simulink model "Road monito-2024r"  (R2021a)
settings: Solver=FixedStepDiscrete  StartTime=0.0  StopTime=inf  FixedStep=0.1  RelTol=1e-3
libraries: simulink x29
(part 1 of 2)
settings Model: Creator=lenovo  LastModifiedBy=lenovo
settings OptimizationCC: DefaultParameterBehavior=Inlined  EnhancedBackFolding=on  PassReuseOutputArgsAs=Individual arguments  ZeroExternalMemoryAtStartup=off  ZeroInternalMemoryAtStartup=off  OptimizeBlockOrder=speed  DifferentSizesBufferReuse=on  OptimizationCustomize=off  EfficientTunableParamExpr=on
settings DebuggingCC: ParameterTunabilityLossMsg=error
settings SFSimCC: MATLABDynamicMemAlloc=off
settings RTWCC: SystemTargetFile=ert.tlc  GenCodeOnly=on  PackageName=VM  TemplateMakefile=ert_default_tmf  GenerateReport=on  Toolchain=Microsoft Visual C++ 2019 v16.0 | nmake (64-bit Windows)  LaunchReport=on  TargetLang=C++
settings CodeAppCC: ForceParamTrailComments=on  IgnoreCustomStorageClasses=off  OperatorAnnotations=on  SimulinkDataObjDesc=on  SFDataObjDesc=on  InsertBlockDesc=on
settings ERTTargetCC: TargetLangStandard=C++03 (ISO)  GenerateSampleERTMain=on  CodeInterfacePackaging=C++ class  SupportContinuousTime=on  SupportVariableSizeSignals=on  InlinedParameterPlacement=NonHierarchical  RootIOFormat=Structure reference  ERTCustomFileTemplate=example_file_process.tlc

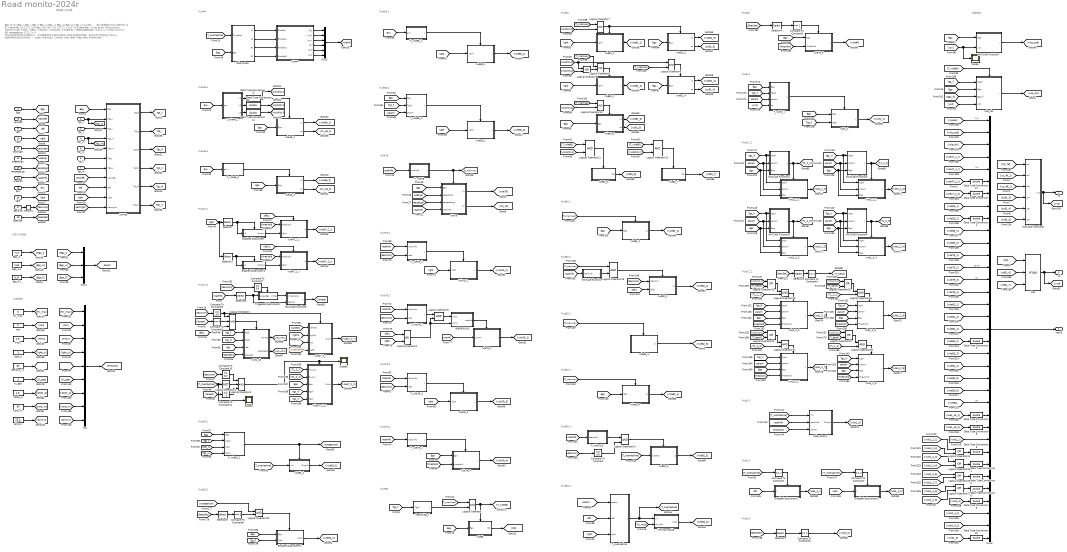
== system Road monito-2024r ==
  note: 法规阈值
  note: 自车几何参数
  note: Rule79.2
  note: Rule79.1
  note: Rule46.2
  note: 信息输入及处理
  note: Rule53.1
  note: Rule78
  note: Rule46.1
  note: Rule53.2
  note: Rule79.4
  note: Rule80
  note: Rule82.2
  note: Rule44
  note: Rule79.3
  note: Rule1.5
  note: Rule1.4
  note: Rule82.4
  note: Rule1.2.1
  note: Rule1.2.2
  note: Rule81
  note: Rule84
  note: Rule82.3
  note: Rule47.2
  note: Rule82.4
  note: Rule58.2
  note: Rule47.1
  note: Ego: [1 7]; [Ego_x Ego_y Ego_h Ego_vx Ego_vy Ego_ax Ego_ay]
      | Tgt_xx: [1 20]; 输入速度单位m/s
      | laneline: [1 6]; [identifier C3 C2 C1 C0 type] y = C3x^3 + C2x^2 + C1x +C0
      | identifier: -1(not exist) 0(Occlusion) 1(exist)
      | type: 1实线，2虚线，3双实线，4左实右虚，5左虚右实，6路肩
      | speedsign: [1 4]; [x y vxmax vxmin = 60]
      | respeedsign: [1 2]; [x y]
      | 自车坐标系原点位于后轴中心，所以需要自车长宽及后轴中心到自车前轴的距离；他车坐标为矩形的几何中心
      | roadinfo:[type,ID,Num]； type:1 mainway, 2 ramp, 3 acc lane, 4 dec lane, 5 eme lane
      | ID:自车所在的车道id，各类型均为最左侧车道id为1，往右递增；
      | Num:同类型同方向车道数
      | Env:[visibility, slip, night]；visibility能见度，slip高滑移路面标识符(1true，0false)，night夜间标识符
      | light:[left, right, fog, far, near, position, front, rear, waring] 均为标识符
      | decision:行为决策信息：1向左换道，2向右换道，3超车，4停车，5倒车，6掉头
      | SpecSec:[bend, tunnel, construction, diversion, merge, mergefollow]；
      | bend弯道路段，tunnel隧道路段，construction施工路段，diversion导流区域，merge合并路段区域，mergefollow合并路段后的区域；(overlap即为进入）
  note: Rule58.1
  note: 结果输出
  note: Rule82.1
  note: Rule82.6
  note: Rule1.3
  note: Rule1.1
  Ego : Inport  PortDimensions=[1 7]
  Tgt_x : Inport  Port=2  PortDimensions=[1 20]
  Tgt_y : Inport  Port=3  PortDimensions=[1 20]
  Tgt_vx : Inport  Port=4  PortDimensions=[1 20]
  Tgt_vy : Inport  Port=5  PortDimensions=[1 20]
  Tgt_l : Inport  Port=6  PortDimensions=[1 20]
  Tgt_w : Inport  Port=7  PortDimensions=[1 20]
  nextleft : Inport  Port=8  PortDimensions=[1 6]
  left : Inport  Port=9  PortDimensions=[1 6]
  right : Inport  Port=10  PortDimensions=[1 6]
  nextright : Inport  Port=11  PortDimensions=[1 6]
  speedsign : Inport  Port=12  PortDimensions=[1 4]
  respeedsign : Inport  Port=13  PortDimensions=[1 2]
  roadinfo : Inport  Port=14  PortDimensions=[1 3]
  Env : Inport  Port=15  PortDimensions=[1 3]
  light : Inport  Port=16  PortDimensions=[1 9]
  decision : Inport  Port=17  PortDimensions=[1 1]
  SpecSec : Inport  Port=18  PortDimensions=[1 6]
  Compare To Constant{,7..8,10} (4 alike) : simulink/Logic and Bit Operations/Compare To Constant  relop===  const=3.0  OutDataTypeStr=boolean
  Compare To Constant{1,3..6} (5 alike) : simulink/Logic and Bit Operations/Compare To Constant  relop===  const=1  OutDataTypeStr=boolean
  Compare To Constant11 : simulink/Logic and Bit Operations/Compare To Constant  relop===  const=-1  OutDataTypeStr=boolean
  Compare To Constant2 : simulink/Logic and Bit Operations/Compare To Constant  relop===  const=2  OutDataTypeStr=boolean
  Compare To Constant9 : simulink/Logic and Bit Operations/Compare To Constant  relop===  const=0  OutDataTypeStr=boolean
  Data Type Conversion{,1..14} (15 alike) : DataTypeConversion  OutDataTypeStr=double
  Ego_fl1 : Constant  Value=6.24
  Ego_l1 : Constant  Value=7.27
  Ego_w1 : Constant  Value=2.55
  Enabled Subsystem : Subsystem  TreatAsAtomicUnit=on
  Enabled Subsystem1 : Subsystem  TreatAsAtomicUnit=on
  Enabled Subsystem2 : Subsystem  TreatAsAtomicUnit=on
  Enabled Subsystem3 : Subsystem  TreatAsAtomicUnit=on
  Enabled Subsystem4 : Subsystem  TreatAsAtomicUnit=on
  Logical Operator{,5,7..18,23} (15 alike) : Logic  AllPortsSameDT=off  OutDataTypeStr=boolean
  Logical Operator1 : Logic  Inputs=3  AllPortsSameDT=off  OutDataTypeStr=boolean
  Logical Operator{2,6,19..22,24..27} (10 alike) : Logic  Operator=OR  AllPortsSameDT=off  OutDataTypeStr=boolean
  Logical Operator3 : Logic  Inputs=3  AllPortsSameDT=off  OutDataTypeStr=boolean
  Logical Operator4 : Logic  Operator=NOT  AllPortsSameDT=off  OutDataTypeStr=boolean
  MATLAB Function : MATLAB Function  TreatAsAtomicUnit=on
  MATLAB Function1 : MATLAB Function  TreatAsAtomicUnit=on
  MATLAB Function2 : MATLAB Function  TreatAsAtomicUnit=on
  MATLAB Function3 : MATLAB Function  TreatAsAtomicUnit=on
  MATLAB Function4 : MATLAB Function  TreatAsAtomicUnit=on
  MATLAB Function5 : MATLAB Function  TreatAsAtomicUnit=on
  MATLAB Function6 : MATLAB Function  TreatAsAtomicUnit=on
  MATLAB Function7 : MATLAB Function  TreatAsAtomicUnit=on
  Max : MinMax  Function=max  Inputs=3
  Memory : Memory
  Mux : Mux  Inputs=9
  Mux1 : Mux  Inputs=3
  Mux2 : Mux  Inputs=6
  Mux3 : Mux  Inputs=35
  Scope : Scope
  Scope2 : Scope
  Scope4 : Scope
  Selector : Selector  InputPortWidth=9  IndexOptions=Index vector (dialog)  Indices=[1]  OutputSizes=1
  Selector1 : Selector  InputPortWidth=9  IndexOptions=Index vector (dialog)  Indices=[2]  OutputSizes=1
  Selector2 : Selector  InputPortWidth=6  IndexOptions=Index vector (dialog)  Indices=[4]  OutputSizes=1
  Selector3 : Selector  InputPortWidth=6  IndexOptions=Index vector (dialog)  Indices=[1]  OutputSizes=1
  Selector4 : Selector  InputPortWidth=6  IndexOptions=Index vector (dialog)  Indices=[3]  OutputSizes=1
  Selector5 : Selector  InputPortWidth=6  IndexOptions=Index vector (dialog)  Indices=[5]  OutputSizes=1
  Selector6 : Selector  InputPortWidth=3  IndexOptions=Index vector (dialog)  Indices=[2]  OutputSizes=1
  Subsystem : Subsystem
  Subsystem2 : Subsystem
  TTCx : Constant  Value=1.8
  T_overlapline : MATLAB Function  TreatAsAtomicUnit=on
  T_rule1_1 : MATLAB Function  TreatAsAtomicUnit=on
  T_rule46_1 : MATLAB Function  TreatAsAtomicUnit=on
  T_rule46_2 : MATLAB Function  TreatAsAtomicUnit=on
  T_rule53_1 : MATLAB Function  TreatAsAtomicUnit=on
  T_rule58_1 : MATLAB Function  TreatAsAtomicUnit=on
  T_rule58_2 : MATLAB Function  TreatAsAtomicUnit=on
  T_rule78 : MATLAB Function  TreatAsAtomicUnit=on
  T_rule79_1 : MATLAB Function  TreatAsAtomicUnit=on
  T_rule79_2 : MATLAB Function  TreatAsAtomicUnit=on
  T_rule79_3 : MATLAB Function  TreatAsAtomicUnit=on
  T_rule79_4 : MATLAB Function  TreatAsAtomicUnit=on
  T_rule79_5 : MATLAB Function  TreatAsAtomicUnit=on
  Timing module : Subsystem
  Triggered Subsystem2 : Subsystem  TreatAsAtomicUnit=on
  cl_gap : Constant  Value=3
  cons_vx : Constant  Value=80
  dclmin : Constant  Value=[-3.4 13.6]
  declane_vx : Constant  Value=60
  isexistTgt_f : MATLAB Function  TreatAsAtomicUnit=on
  latdis_p : Constant  Value=1.8
  light_cl : Constant  Value=3
  nan : Constant  Value=0
  rule1_1 : Subsystem  TreatAsAtomicUnit=on
  rule1_2_1 : Subsystem  TreatAsAtomicUnit=on
  rule1_2_2 : Subsystem  TreatAsAtomicUnit=on
  rule1_2_3 : Subsystem  TreatAsAtomicUnit=on
  rule1_2_4 : Subsystem  TreatAsAtomicUnit=on
  rule1_2_5 : Subsystem  TreatAsAtomicUnit=on
  rule1_2_6 : Subsystem  TreatAsAtomicUnit=on
  rule1_2_7 : Subsystem  TreatAsAtomicUnit=on
  rule1_2_8 : Subsystem  TreatAsAtomicUnit=on
  rule1_43 : Subsystem  TreatAsAtomicUnit=on
  rule44 : Subsystem
  rule46_1 : Subsystem  TreatAsAtomicUnit=on
  rule46_2 : Subsystem  TreatAsAtomicUnit=on
  rule47_1_l : Subsystem  TreatAsAtomicUnit=on
  rule47_1_r : Subsystem  TreatAsAtomicUnit=on
  rule47_2_r : Subsystem  TreatAsAtomicUnit=on
  rule53_1 : Subsystem  TreatAsAtomicUnit=on
  rule58_1 : Subsystem  TreatAsAtomicUnit=on
  rule58_2 : Subsystem  TreatAsAtomicUnit=on
  rule78 : Subsystem  TreatAsAtomicUnit=on
  rule79_1 : Subsystem  TreatAsAtomicUnit=on
  rule79_2 : Subsystem  TreatAsAtomicUnit=on
  rule79_3 : Subsystem  TreatAsAtomicUnit=on
  rule79_4 : Subsystem  TreatAsAtomicUnit=on
  rule79_5 : Subsystem  TreatAsAtomicUnit=on
  rule80 : Subsystem  TreatAsAtomicUnit=on
  rule81_1 : Subsystem  TreatAsAtomicUnit=on
  rule81_2 : Subsystem  TreatAsAtomicUnit=on
  rule81_3 : Subsystem  TreatAsAtomicUnit=on
  rule81_4 : Subsystem  TreatAsAtomicUnit=on
  rule81_5 : Subsystem  TreatAsAtomicUnit=on
  rule81_6 : Subsystem  TreatAsAtomicUnit=on
  rule81_7 : Subsystem  TreatAsAtomicUnit=on
  rule82_1 : Subsystem  TreatAsAtomicUnit=on
  rule82_2 : Subsystem  TreatAsAtomicUnit=on
  rule82_3 : Subsystem  TreatAsAtomicUnit=on
  rule82_4 : Subsystem  TreatAsAtomicUnit=on
  rule82_5 : Subsystem  TreatAsAtomicUnit=on
  rule_47_2_2 : Subsystem  TreatAsAtomicUnit=on
  rule_dis : Subsystem  TreatAsAtomicUnit=on
  tcl_max : Constant  Value=6
  zoning : MATLAB Function  TreatAsAtomicUnit=on
  使能信号生成 : Subsystem
  result : Outport
  cs : Outport  Port=2
  cd : Outport  Port=3
  tag scope: Ego=global, Env=global, Tgt_f=global, Tgt_lf=global, Tgt_lr=global, Tgt_r=global, Tgt_rf=global, Tgt_rr=global, left=global, light=global, nextleft=global, nextright=global, param=global, respdsign=global, right=global, roadinfo=global, spdsign=global, threshold=global
  wires:
  [T_mainway] -> rule82_4/Enable
  Selector3/1 -> Compare To Constant4/1
  [rule47_1_l] -> Mux3/4
  Logical Operator24/1 -> Data Type Conversion3/1
  [roadinfo] -> Selector6/1
  [Ego] -> rule1_2_5/3(Ego)
  rule81_3/2(cs) -> [cs81_3]
  Ego_w1/1 -> [Ego_w]
  [T1_2_2] -> Logical Operator16/2
  rule81_1/1(y) -> [rule81_1]
  [T1_2_3] -> Logical Operator17/2
  rule1_2_1/1(y) -> [rule1_2_1]
  Logical Operator15/1 -> rule1_2_5/Enable
  [laneot] -> Compare To Constant11/1
  Data Type Conversion7/1 -> Mux3/25
  [rule1_2_3] -> Logical Operator24/2
  [Tgt_f] -> isexistTgt_f/1(Tgt_f)
  [T_mainway] -> Logical Operator9/2
  Enabled Subsystem4/1(Out2) -> [rule53_2]
  MATLAB Function5/1(y) -> [laneot]
  Tgt_vx/1 -> [Tgt_vx], zoning/4(Tgt_vx)
  rule47_1_r/1(y1) -> [rule47_1_r]
  TTCx/1 -> [TTCx]
  Selector4/1 -> Compare To Constant5/1
  Logical Operator19/1 -> Logical Operator15/1
  [Ego_l] -> Mux1/1
  [rule1_5] -> Data Type Conversion10/1
  [Ego_fl] -> Mux1/3
  [Visibility1] -> Logical Operator19/1
  T_rule1_1/1(y) -> rule1_1/Enable
  [rule_spd] -> Mux3/2
  [SpecSec] -> Selector2/1
  [light] -> rule81_1/1(light)
  [rule1_2_2] -> Logical Operator25/1
  Logical Operator21/1 -> Logical Operator17/1
  [nan] -> Mux/2
  Selector6/1 -> MATLAB Function5/2(laneid), Triggered Subsystem2/1(lane_Ego)
  Data Type Conversion6/1 -> Mux3/31
  T_rule79_5/1(y) -> Logical Operator14/1
  Enabled Subsystem3/1(y) -> [rule1_4_2]
  Logical Operator26/1 -> Data Type Conversion5/1
  [param] -> T_rule1_1/3(param)
  rule79_5/1(y) -> [rule84]
  rule81_5/1(y1) -> [rule81_5]
  [CD] -> Max/1
  Data Type Conversion10/1 -> Mux3/35
  [T_bend] -> Logical Operator20/2
  [rule81_1] -> Mux3/16
  Triggered Subsystem2/1(initial) -> MATLAB Function5/1(initiallane)
  nan/1 -> [nan]
  [T_bend] -> Logical Operator22/2
  [Ego] -> rule81_4/1(Ego)
  Compare To Constant2/1 -> Enabled Subsystem3/Enable
  [light] -> rule58_1/1(light)
  Subsystem/4(R2) -> rule44/4(Enable3)
  Logical Operator9/1 -> rule81_4/Enable
  rule82_2/1(y1) -> [rule82_2]
  Compare To Constant11/1 -> Logical Operator3/3
  Mux/1 -> [threshold]
  [T_overlapline] -> Subsystem2/1(In1)
  [left2] -> Logical Operator2/2
  [light] -> rule58_2/1(light)
  left/1 -> [left]
  [roadinfo] -> rule78/4(roadinfo)
  [rule1_43_1] -> Data Type Conversion7/1
  [threshold] -> Subsystem2/3(param)
  使能信号生成/1(enable) -> rule79_2/Enable
  [SpecSec] -> rule1_43/4(specsec)
  T_rule46_2/1(y) -> rule46_2/Enable
  rule46_1/1(y1) -> [rule46_1]
  Logical Operator7/1 -> rule81_3/Enable, rule81_1/Enable
  [threshold] -> rule1_2_8/4(threshold)
  rule79_1/1(y) -> [rule79_1]
  Mux3/1 -> result/1
  [rule53_2] -> Data Type Conversion1/1
  rule81_3/1(y1) -> [rule81_3]
  tcl_max/1 -> [Tcl_max]
  Data Type Conversion8/1 -> Mux3/26
  Tgt_w/1 -> zoning/7(Tgt_w)
  [Ego] -> rule1_2_6/3(Ego)
  Subsystem/1(L1) -> rule44/1(Enable)
  rule82_5/1(y1) -> [rule82_5]
  Logical Operator1/1 -> rule1_43/Enable
  [rule82_6] -> Mux3/23
  Enabled Subsystem1/1(Output) -> rule47_1_r/2(light)
  [decision] -> Compare To Constant7/1
  [light] -> rule79_1/1(light)
  rule1_2_2/1(y) -> [rule1_2_2]
  [CS_78] -> MATLAB Function6/1(cs1)
  [left1] -> Logical Operator1/3
  [Visibility1] -> Logical Operator21/1
  rule82_4/1(y1) -> [rule82_4]
  [threshold] -> rule47_1_r/1(threshold)
  [decision] -> Compare To Constant10/1
  Logical Operator22/1 -> Logical Operator18/1
  [Ego_w] -> Mux1/2
  [cd81_7] -> Max/3
  [Tgt_lf] -> rule1_43/2(Tgtlf)
  right/1 -> [right]
  [right] -> zoning/10(right)
  [Ego] -> T_rule1_1/1(Ego)
  [rule53_1] -> Mux3/8
  [Ego] -> rule81_5/1(Ego)
  [T_mainway] -> Logical Operator13/1
  [Ego] -> rule_dis/2(Ego)
  [cl_gap] -> Mux/6
  [Ego] -> rule82_1/1(Ego)
  [congestion] -> Logical Operator23/1
  [left] -> Enabled Subsystem2/1(u)
  Ego_fl1/1 -> [Ego_fl]
  Tgt_l/1 -> zoning/6(Tgt_l)
  [left] -> rule1_43/3(left)
  rule58_1/1(y) -> [rule58_1]
  T_overlapline/1(y) -> [T_overlapline], Timing module/1(y1)
  rule44/4(cl_f) -> Mux2/4
  rule47_1_l/1(y1) -> [rule47_1_l]
  rule58_2/1(y) -> [rule58_2]
  Logical Operator3/1 -> rule_47_2_2/Enable, Scope2/1
  [T_mainway] -> Logical Operator8/1
  [param] -> MATLAB Function4/2(param), rule1_2_4/2(param)
  [Visibility1] -> Logical Operator10/2
  zoning/4(Tgt_lr) -> [Tgt_lr]
  [cs81_4] -> MATLAB Function6/5(cs5)
  [light] -> rule79_3/1(light)
  [ycd] -> rule_dis/4(ycd)
  [Ego] -> rule1_2_2/3(Ego), MATLAB Function2/3(Ego)
  [threshold] -> rule79_4/2(threshold)
  [roadinfo] -> T_rule78/1(roadinfo)
  T_rule53_1/1(y) -> rule53_1/Enable, [congestion]
  Logical Operator10/1 -> rule81_5/Enable
  [T_overlapline] -> rule53_1/1(In1)
  [rule1_4_1] -> Mux3/33
  respeedsign/1 -> [respdsign]
  Mux1/1 -> [param]
  Logical Operator23/1 -> Enabled Subsystem4/Enable
  [T_mainway] -> Logical Operator/1
  rule44/3(cr_rr) -> Mux2/3
  [Tgt_rf] -> rule1_2_8/1(Tgtrr)
  [left1] -> rule47_2_r/4(left1)
  [T_mainway] -> Logical Operator10/1
  [declane_vx] -> Mux/5
  cl_gap/1 -> [cl_gap]
  [T_rule80] -> Logical Operator11/1
  [Ego] -> rule79_4/1(Ego)
  rule81_2/1(y) -> [rule81_2]
  [cs81_5] -> MATLAB Function6/6(cs6)
  [Ego] -> T_rule53_1/1(Ego)
  [Ego_fl] -> rule_dis/3(Ego_fl)
  [T1_2_4] -> Logical Operator18/2
  rule79_2/1(y) -> [rule79_2]
  speedsign/1 -> [spdsign]
  [roadinfo] -> MATLAB Function/1(roadinfo)
  zoning/3(Tgt_lf) -> [Tgt_lf]
  [rule44] -> Mux3/1  "1-6"
  [T_overlapline] -> Compare To Constant1/1
  [right] -> Enabled Subsystem3/1(u)
  [Ego] -> rule1_2_8/3(Ego)
  Logical Operator25/1 -> Data Type Conversion4/1
  nextleft/1 -> [nextleft]
  [rule1_2_6] -> Logical Operator27/1
  Compare To Constant10/1 -> Logical Operator3/1
  rule1_2_5/1(y) -> [rule1_2_5]
  [Tgt_rr] -> MATLAB Function4/1(Tgtrr), rule1_2_4/1(Tgtrr)
  rule79_3/1(y) -> [rule79_3]
  [rule79_3] -> Mux3/14  "20"
  Memory/1 -> [decision]
  [roadinfo] -> T_rule79_5/1(roadinfo)
  [rule1_4_2] -> Mux3/34
  [light_cl] -> Mux/4
  [param] -> rule1_2_8/2(param)
  rule78/2(y2) -> [CS_78]
  Logical Operator20/1 -> Logical Operator16/1
  [rule1_2_1] -> Logical Operator24/1
  [T1_2_1] -> Logical Operator15/2
  latdis_p/1 -> [latdis_p]
  decision/1 -> Memory/1
  [left] -> T_overlapline/2(left)
  Enabled Subsystem/1(Output) -> rule47_1_l/2(light)
  [Ego] -> rule1_1/1(Ego)
  [param] -> T_rule58_2/3(param)
  rule53_1/1(Output) -> [rule53_1]
  rule79_4/1(y) -> [rule79_4]
  Subsystem/3(R1) -> rule44/3(Enable2)
  [roadinfo] -> T_rule79_3/1(roadinfo)
  [Ego] -> MATLAB Function4/3(Ego), rule1_2_4/3(Ego)
  [TTCx] -> Mux/3
  Selector5/1 -> Compare To Constant6/1
  [T1_2_4] -> rule_47_2_2/2(t1_2_4)
  [Ego] -> rule46_1/1(Ego)
  rule81_4/1(y1) -> [rule81_4]
  [light] -> rule81_2/1(light)
  [decision] -> T_rule79_3/2(dec)
  [Visibility1] -> Logical Operator6/2
  [rule82_1] -> Mux3/18
  rule46_2/2(cs) -> [cs_46_2]
  [rule84] -> Mux3/24  "30"
  Compare To Constant7/1 -> Triggered Subsystem2/Trigger
  rule46_2/1(y1) -> [rule46_2]
  [Ego] -> zoning/1(Ego)
  Tgt_vy/1 -> zoning/5(Tgt_vy)
  T_rule58_1/1(y) -> rule58_1/Enable
  [rule82_2] -> Data Type Conversion2/1
  [T_rule80] -> rule_dis/Enable
  [Tgt_rf] -> rule1_2_2/1(Tgtrf), MATLAB Function2/1(Tgtrf)
  [nextleft] -> zoning/8(nextleft)
  [roadinfo] -> T_rule79_2/1(roadinfo)
  [rule1_2_7] -> Logical Operator26/2
  Enabled Subsystem2/1(y) -> [rule1_4_1]
  Tgt_x/1 -> [Tgt_x], zoning/2(Tgt_x)
  [cd81_6] -> Max/2
  [rule47_1_r] -> Mux3/5  "10"
  [T_overlapline] -> rule82_5/1(overlap)
  [respdsign] -> rule78/3(respeedsign)
  [T_bend] -> Logical Operator21/2
  [Tgt_x] -> T_rule53_1/3(Tgtx)
  [rule81_2] -> Mux3/17
  Logical Operator12/1 -> rule81_7/Enable
  Data Type Conversion9/1 -> Mux3/32
  [Tgt_rr] -> rule_47_2_2/5(Tgtrr)
  [rule82_3] -> Mux3/20
  Env/1 -> [Env]
  [cons_vx] -> Mux/8
  [param] -> rule1_2_3/2(param), MATLAB Function3/2(param)
  [rule58_1] -> Mux3/10
  [Tgt_rf] -> rule_47_2_2/4(Tgtrf)
  Data Type Conversion4/1 -> Mux3/29
  [rule79_1] -> Mux3/12
  [rule47_2_r] -> Data Type Conversion11/1
  [Tgt_vx] -> T_rule53_1/4(Tgtvx)
  [rule1_1] -> Mux3/27
  T_rule46_1/1(y1) -> Data Type Conversion12/1
  Timing module/1(Out2) -> [rule82_6]
  isexistTgt_f/1(y) -> Logical Operator/2
  rule78/1(y1) -> [rule78]
  MATLAB Function2/1(y) -> [T1_2_2], rule1_2_2/Enable
  [Tgt_f] -> rule_dis/1(Tgt_f)
  [Ego] -> rule1_2_1/3(Ego), MATLAB Function1/3(Ego)
  Selector/1 -> Enabled Subsystem/1(y1), Enabled Subsystem/Enable
  [right1] -> rule47_2_r/2(right1)
  [Tgt_f] -> rule1_1/2(Tgtf)
  [param] -> T_overlapline/1(param)
  [left1] -> rule82_2/2(left1)
  Logical Operator16/1 -> rule1_2_6/Enable
  [latdis_p] -> Mux/7
  [threshold] -> rule79_5/2(threshold)
  [Tgt_rf] -> rule1_2_6/1(Tgtrf)
  [param] -> rule1_2_7/2(param)
  [rule47_2_2] -> Data Type Conversion/1
  [Ego] -> rule79_5/1(Ego)
  declane_vx/1 -> [declane_vx]
  Logical Operator18/1 -> rule1_2_8/Enable
  T_rule79_2/1(y) -> Logical Operator5/1
  [Visibility1] -> Logical Operator22/1
  [param] -> rule1_2_6/2(param)
  MATLAB Function4/1(y) -> rule1_2_4/Enable, [T1_2_4]
  [Ego] -> rule1_2_3/3(Ego), MATLAB Function3/3(Ego)
  rule1_2_3/1(y) -> [rule1_2_3]
  zoning/1(Tgt_f) -> [Tgt_f]
  [T_bend] -> Logical Operator19/2
  [roadinfo] -> T_rule79_4/1(roadinfo)
  rule82_1/1(y1) -> [rule82_1]
  Logical Operator27/1 -> Data Type Conversion6/1
  [threshold] -> rule1_2_6/4(Threshold)
  Logical Operator5/1 -> 使能信号生成/1(pros)
  [Tgt_f] -> rule1_43/1(Tgtf)
  [Ego] -> T_rule58_2/1(Ego)
  [rule79_4] -> Mux3/15
  Compare To Constant3/1 -> [rule1_5]
  [param] -> rule1_2_2/2(param), MATLAB Function2/2(param)
  [Tgt_f] -> T_rule1_1/2(Tgt_f)
  rule80/1(CD) -> [CD]
  [Ego] -> rule_47_2_2/3(Ego)
  [SpecSec] -> Selector3/1
  rule46_1/2(cs) -> [cs_46_1]
  [right1] -> rule47_1_r/Enable
  Data Type Conversion/1 -> Mux3/7
  SpecSec/1 -> [SpecSec]
  Subsystem2/1(Output) -> [rule1_3]
  Data Type Conversion11/1 -> Mux3/6
  [rule1_2_8] -> Logical Operator27/2
  [rule58_2] -> Mux3/11
  [T_mainway] -> Logical Operator7/1
  Mux2/1 -> [rule44]
  zoning/5(Tgt_rf) -> [Tgt_rf]
  [Tgt_f] -> T_rule53_1/2(Tgt_f)
  [decision] -> T_rule79_1/2(dec)
  [decision] -> T_rule79_2/2(dec)
  roadinfo/1 -> [roadinfo]
  [T_overlapline] -> Compare To Constant2/1
  Logical Operator11/1 -> rule81_6/Enable
  [Ego] -> rule80/1(Ego)
  rule82_3/1(y1) -> [rule82_3]
  [left] -> zoning/9(left)
  Data Type Conversion3/1 -> Mux3/28
  Logical Operator/1 -> rule80/Enable, [T_rule80]
  rule1_1/1(y) -> [rule1_1]
  [T_overlapline] -> rule47_2_r/3(Tol)
  MATLAB Function3/1(y) -> rule1_2_3/Enable, [T1_2_3]
  [rule44] -> rule79_2/1(rule44)
  rule1_2_7/1(y) -> [rule1_2_7]
  [roadinfo] -> T_rule79_1/1(roadinfo)
  [threshold] -> rule1_2_5/4(threshold)
  rule47_2_r/1(Out1) -> [rule47_2_r]
  rule44/6(cl_lr) -> Mux2/6
  Tgt_y/1 -> zoning/3(Tgt_y)
  [Visibility3] -> Logical Operator11/2
  [Ego] -> rule46_2/1(Ego)
  [Tcl_max] -> Mux/1
  [rule1_2_5] -> Logical Operator26/1
  [T_overlapline] -> Scope4/1, Logical Operator4/1
  Logical Operator2/1 -> Logical Operator5/2, 使能信号生成/2(cons)
  zoning/6(Tgt_rr) -> [Tgt_rr]
  [threshold] -> rule1_2_7/4(threshold)
  T_rule79_1/1(y) -> rule79_1/Enable
  [right] -> T_overlapline/3(right)
  Ego_l1/1 -> [Ego_l]
  [decision] -> Compare To Constant8/1
  Logical Operator6/1 -> Logical Operator8/2
  light/1 -> [light]
  [rule82_4] -> Mux3/21
  [cs_46_1] -> MATLAB Function6/2(cs2)
  [light] -> Selector1/1, Selector/1
  T_rule79_3/1(y) -> rule79_3/Enable
  Subsystem/2(L2) -> rule44/2(Enable1)
  [T_overlapline] -> Subsystem/1(Toverlap)
  [rule79_2] -> Mux3/13  "18-19"
  Compare To Constant6/1 -> Logical Operator23/2
  [spdsign] -> rule78/2(speedsign)
  [Ego] -> Subsystem/2(Ego)
  Max/1 -> [ycd], cd/1
  [Ego] -> rule82_4/1(Ego)
  [decision] -> Compare To Constant/1
  MATLAB Function7/1(y) -> [rule_spd]
  MATLAB Function6/1(ycs) -> [ycs], cs/1
  [Env] -> T_rule46_1/1(env)
  MATLAB Function1/1(y) -> rule1_2_1/Enable, [T1_2_1]
  [laneot] -> rule47_2_r/1(laneot)
  [Visibility1] -> Logical Operator20/1
  [param] -> rule1_2_5/2(param)
  [T_mainway] -> rule82_1/Enable
  nextright/1 -> [nextright]
  Compare To Constant5/1 -> rule79_5/Enable
  rule1_2_8/1(y) -> [rule1_2_8]
  [Ego] -> rule1_2_7/3(Ego)
  Compare To Constant4/1 -> [T_bend]
  rule1_2_4/1(y) -> [rule1_2_4]
  Compare To Constant/1 -> Logical Operator14/2
  rule44/2(cr_rf) -> Mux2/2
  rule_47_2_2/1(Out1) -> [rule47_2_2]
  [rule1_43_2] -> Data Type Conversion8/1
  Data Type Conversion2/1 -> Mux3/19
  [Tgt_f] -> T_rule58_2/2(Tgt_f)
  Logical Operator13/1 -> rule82_2/Enable
  [cs81_3] -> MATLAB Function6/4(cs4)
  [Ego] -> Enabled Subsystem4/1(Ego)
  Logical Operator17/1 -> rule1_2_7/Enable
  [param] -> rule1_2_1/2(param), MATLAB Function1/2(param)
  MATLAB Function/1(y) -> Logical Operator13/2
  light_cl/1 -> [light_cl]
  zoning/2(Tgt_r) -> [Tgt_r]
  [rule82_5] -> Mux3/22
  [Tgt_lr] -> rule1_2_3/1(Tgtlr), MATLAB Function3/1(Tgtlr)
  [Visibility3] -> Logical Operator7/2
  T_rule78/1(y) -> [T_mainway], rule78/Enable
  [Tgt_lr] -> rule1_2_7/1(Tgtlr)
  [Visibility2] -> Logical Operator9/1, Logical Operator6/1
  [ycs] -> Scope/1, MATLAB Function7/2(ycs)
  [Tcl_max] -> Timing module/2(tcl_max)
  rule81_7/1(CD) -> [cd81_7]
  Selector1/1 -> Enabled Subsystem1/Enable, Enabled Subsystem1/1(y1)
  [rule1_3] -> Data Type Conversion9/1
  [Env] -> T_rule46_2/1(env)
  [T_mainway] -> rule82_3/Enable
  rule44/5(cl_lf) -> Mux2/5
  [rule1_2_4] -> Logical Operator25/2
  [Ego] -> MATLAB Function7/1(Ego)
  [Tgt_lf] -> rule1_2_1/1(Tgtlf), MATLAB Function1/1(Tgtlf)
  [cs_46_2] -> MATLAB Function6/3(cs3)
  rule81_6/1(CD) -> [cd81_6]
  [Visibility2] -> Logical Operator12/2
  rule44/1(cr_f) -> Mux2/1
  [T1_2_2] -> rule_47_2_2/1(T1_2_2)
  [roadinfo] -> Subsystem2/2(roadinfo)
  Data Type Conversion1/1 -> Mux3/9
  [SpecSec] -> Selector4/1
  Ego/1 -> [Ego]
  [left1] -> Logical Operator2/1
  Compare To Constant8/1 -> rule47_2_r/Enable, Logical Operator1/1
  rule1_43/2(specsecot) -> [rule1_43_2]
  rule1_2_6/1(y) -> [rule1_2_6]
  [Tgt_lf] -> rule1_2_5/1(Tgtlf)
  [decision] -> rule82_2/1(decision)
  Logical Operator4/1 -> Logical Operator3/2
  [Ego] -> rule81_3/1(Ego)
  rule81_5/2(cs) -> [cs81_5]
  [Tgt_f] -> Enabled Subsystem4/2(Tgtf)
  Compare To Constant9/1 -> Logical Operator1/2
  T_rule79_4/1(y) -> rule79_4/Enable
  [threshold] -> rule47_1_l/1(threshold)
  Compare To Constant1/1 -> Enabled Subsystem2/Enable
  [nextright] -> zoning/11(nextright)
  Data Type Conversion5/1 -> Mux3/30
  [Ego] -> rule78/1(Ego)
  rule_dis/1(y) -> [rule_dis]
  Logical Operator8/1 -> rule81_2/Enable
  Selector2/1 -> Compare To Constant3/1
  [rule_dis] -> Mux3/3
  [ycs] -> T_rule1_1/4(cs)
  [SpecSec] -> Selector5/1
  [left1] -> rule47_1_l/Enable
  cons_vx/1 -> [cons_vx]
  Logical Operator14/1 -> rule82_5/Enable
  rule1_43/1(frontot) -> [rule1_43_1]
  [Env] -> T_rule58_1/1(env)
  T_rule58_2/1(y) -> rule58_2/Enable
  [T_rule80] -> Logical Operator12/1
  [laneot] -> Compare To Constant9/1
  rule81_4/2(cs) -> [cs81_4]
  Data Type Conversion12/1 -> rule46_1/Enable, [Visibility1]
  T_rule46_1/2(y2) -> Data Type Conversion13/1
  Data Type Conversion13/1 -> [Visibility2]
  T_rule46_1/3(y3) -> Data Type Conversion14/1
  Data Type Conversion14/1 -> [Visibility3]
  dclmin/1 -> [dclmin]
  [dclmin] -> Mux/9

== system Road monito-2024r/Enabled Subsystem ==
  y1 : Inport
  Enable : EnablePort  StatesWhenEnabling=reset
  Add : Sum  Inputs=-+
  Clock3 : Clock
  Constant : Constant  Value=0
  Memory : Memory
  Memory1 : Memory
  Min : MinMax  Function=max  Inputs=2
  Triggered Subsystem2 : Subsystem  TreatAsAtomicUnit=on
  Output : Outport  OutputWhenDisabled=reset  InitialOutput=0
  wires:
  Clock3/1 -> Memory1/1
  y1/1 -> Memory/1
  Triggered Subsystem2/1(Output) -> Add/1
  Memory/1 -> Triggered Subsystem2/Trigger
  Memory1/1 -> Add/2, Triggered Subsystem2/1(In1)
  Min/1 -> Output/1
  Add/1 -> Min/1
  Constant/1 -> Min/2

== system Road monito-2024r/Enabled Subsystem1 ==
  y1 : Inport
  Enable : EnablePort  StatesWhenEnabling=reset
  Add : Sum  Inputs=-+
  Clock3 : Clock
  Constant : Constant  Value=0
  Memory : Memory
  Memory1 : Memory
  Min : MinMax  Function=max  Inputs=2
  Triggered Subsystem2 : Subsystem  TreatAsAtomicUnit=on
  Output : Outport  OutputWhenDisabled=reset  InitialOutput=0
  wires:
  Constant/1 -> Min/2
  Add/1 -> Min/1
  Min/1 -> Output/1
  Memory1/1 -> Triggered Subsystem2/1(In1), Add/2
  Memory/1 -> Triggered Subsystem2/Trigger
  Triggered Subsystem2/1(Output) -> Add/1
  y1/1 -> Memory/1
  Clock3/1 -> Memory1/1

== system Road monito-2024r/Enabled Subsystem2 ==
  u : Inport
  Enable : EnablePort
  MATLAB Function : MATLAB Function  TreatAsAtomicUnit=on
  y : Outport
  wires:
  u/1 -> MATLAB Function/1(left)
  MATLAB Function/1(y) -> y/1

== system Road monito-2024r/Enabled Subsystem3 ==
  u : Inport
  Enable : EnablePort
  MATLAB Function : MATLAB Function  TreatAsAtomicUnit=on
  y : Outport
  wires:
  u/1 -> MATLAB Function/1(left)
  MATLAB Function/1(y) -> y/1

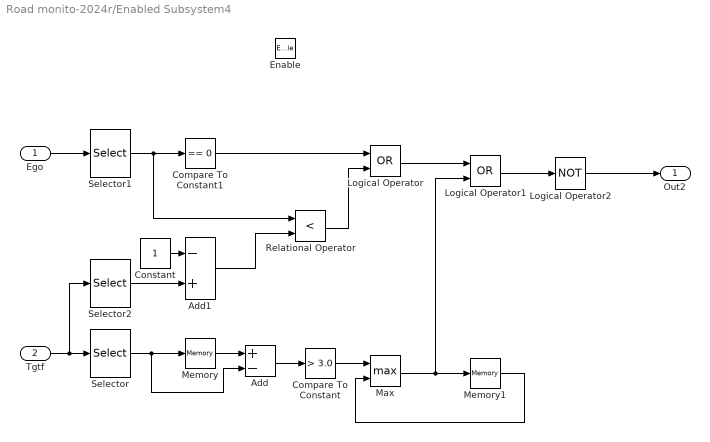
== system Road monito-2024r/Enabled Subsystem4 ==
  Ego : Inport
  Tgtf : Inport  Port=2
  Enable : EnablePort
  Add : Sum  Inputs=+-
  Add1 : Sum  Inputs=-+
  Compare To Constant : simulink/Logic and Bit Operations/Compare To Constant  relop=>  const=3.0  OutDataTypeStr=boolean
  Compare To Constant1 : simulink/Logic and Bit Operations/Compare To Constant  relop===  const=0  OutDataTypeStr=boolean
  Constant : Constant
  Logical Operator : Logic  Operator=OR  AllPortsSameDT=off  OutDataTypeStr=boolean
  Logical Operator1 : Logic  Operator=OR  AllPortsSameDT=off  OutDataTypeStr=boolean
  Logical Operator2 : Logic  Operator=NOT  AllPortsSameDT=off  OutDataTypeStr=boolean
  Max : MinMax  Function=max  Inputs=2
  Memory : Memory  InheritSampleTime=on
  Memory1 : Memory
  Relational Operator : RelationalOperator  Operator=<  OutDataTypeStr=boolean  RndMeth=Simplest
  Selector : Selector  InputPortWidth=6  IndexOptions=Index vector (dialog)  Indices=[1]  OutputSizes=1
  Selector1 : Selector  InputPortWidth=7  IndexOptions=Index vector (dialog)  Indices=[4]  OutputSizes=1
  Selector2 : Selector  InputPortWidth=6  IndexOptions=Index vector (dialog)  Indices=[3]  OutputSizes=1
  Out2 : Outport
  wires:
  Selector/1 -> Add/2, Memory/1
  Add/1 -> Compare To Constant/1
  Memory/1 -> Add/1
  Tgtf/1 -> Selector2/1, Selector/1
  Memory1/1 -> Max/2
  Max/1 -> Logical Operator1/2, Memory1/1
  Compare To Constant/1 -> Max/1
  Ego/1 -> Selector1/1
  Selector1/1 -> Relational Operator/1, Compare To Constant1/1
  Selector2/1 -> Add1/2
  Constant/1 -> Add1/1
  Add1/1 -> Relational Operator/2
  Compare To Constant1/1 -> Logical Operator/1
  Relational Operator/1 -> Logical Operator/2
  Logical Operator/1 -> Logical Operator1/1
  Logical Operator1/1 -> Logical Operator2/1
  Logical Operator2/1 -> Out2/1

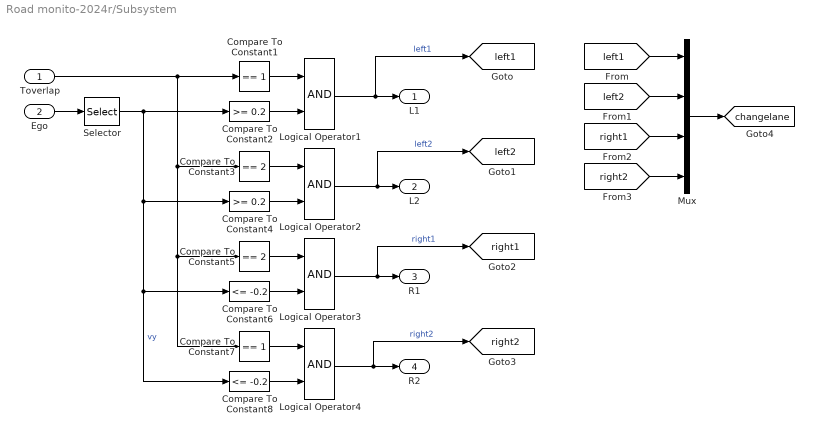
== system Road monito-2024r/Subsystem ==
  Toverlap : Inport
  Ego : Inport  Port=2
  Compare To Constant1 : simulink/Logic and Bit Operations/Compare To Constant  relop===  const=1  OutDataTypeStr=boolean
  Compare To Constant2 : simulink/Logic and Bit Operations/Compare To Constant  relop=>=  const=0.2  OutDataTypeStr=boolean
  Compare To Constant3 : simulink/Logic and Bit Operations/Compare To Constant  relop===  const=2  OutDataTypeStr=boolean
  Compare To Constant4 : simulink/Logic and Bit Operations/Compare To Constant  relop=>=  const=0.2  OutDataTypeStr=boolean
  Compare To Constant5 : simulink/Logic and Bit Operations/Compare To Constant  relop===  const=2  OutDataTypeStr=boolean
  Compare To Constant6 : simulink/Logic and Bit Operations/Compare To Constant  relop=<=  const=-0.2  OutDataTypeStr=boolean
  Compare To Constant7 : simulink/Logic and Bit Operations/Compare To Constant  relop===  const=1  OutDataTypeStr=boolean
  Compare To Constant8 : simulink/Logic and Bit Operations/Compare To Constant  relop=<=  const=-0.2  OutDataTypeStr=boolean
  Logical Operator{1..4} (4 alike) : Logic  AllPortsSameDT=off  OutDataTypeStr=boolean
  Mux : Mux
  Selector : Selector  InputPortWidth=7  IndexOptions=Index vector (dialog)  Indices=[5]  OutputSizes=1
  L1 : Outport
  L2 : Outport  Port=2
  R1 : Outport  Port=3
  R2 : Outport  Port=4
  tag scope: changelane=global, left1=global, left2=global, right1=global, right2=global
  wires:
  Toverlap/1 -> Compare To Constant7/1, Compare To Constant5/1, Compare To Constant3/1, Compare To Constant1/1
  Selector/1 -> Compare To Constant4/1, Compare To Constant8/1, Compare To Constant6/1, Compare To Constant2/1  "vy"
  Compare To Constant1/1 -> Logical Operator1/1
  Logical Operator1/1 -> [left1], L1/1  "left1"
  Compare To Constant2/1 -> Logical Operator1/2
  Ego/1 -> Selector/1
  Logical Operator2/1 -> [left2], L2/1  "left2"
  Compare To Constant3/1 -> Logical Operator2/1
  Compare To Constant4/1 -> Logical Operator2/2
  Logical Operator3/1 -> [right1], R1/1  "right1"
  Compare To Constant5/1 -> Logical Operator3/1
  Compare To Constant6/1 -> Logical Operator3/2
  Logical Operator4/1 -> [right2], R2/1  "right2"
  Compare To Constant7/1 -> Logical Operator4/1
  Compare To Constant8/1 -> Logical Operator4/2
  [left1] -> Mux/1
  [left2] -> Mux/2
  [right1] -> Mux/3
  [right2] -> Mux/4
  Mux/1 -> [changelane]

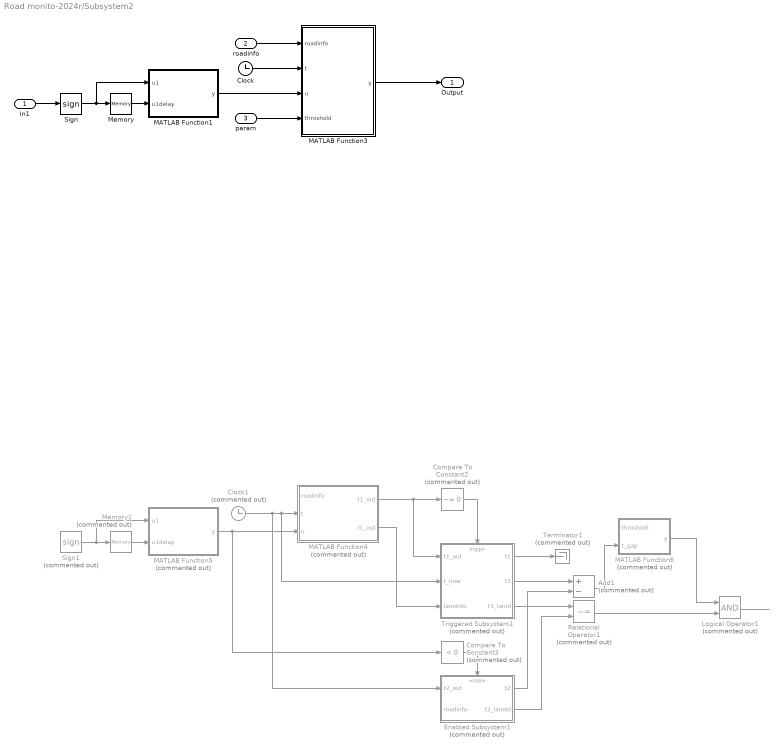
== system Road monito-2024r/Subsystem2 ==
  In1 : Inport
  roadinfo : Inport  Port=2
  param : Inport  Port=3
  Add1 : Sum  Commented=on  Inputs=+-
  Clock : Clock
  Clock1 : Clock  Commented=on
  Compare To Constant2 : simulink/Logic and Bit Operations/Compare To Constant  Commented=on  relop=~=  const=0  OutDataTypeStr=boolean
  Compare To Constant3 : simulink/Logic and Bit Operations/Compare To Constant  Commented=on  relop=<  const=0  OutDataTypeStr=boolean
  Enabled Subsystem1 : Subsystem  Commented=on  TreatAsAtomicUnit=on
  Logical Operator1 : Logic  Commented=on  AllPortsSameDT=off  OutDataTypeStr=boolean
  MATLAB Function1 : MATLAB Function  TreatAsAtomicUnit=on
  MATLAB Function3 : MATLAB Function  TreatAsAtomicUnit=on
  MATLAB Function4 : MATLAB Function  Commented=on  TreatAsAtomicUnit=on
  MATLAB Function5 : MATLAB Function  Commented=on  TreatAsAtomicUnit=on
  MATLAB Function6 : MATLAB Function  Commented=on  TreatAsAtomicUnit=on
  Memory : Memory
  Memory1 : Memory  Commented=on
  Relational Operator1 : RelationalOperator  Commented=on  Operator=~=  OutDataTypeStr=boolean  RndMeth=Simplest
  Sign : Signum
  Sign1 : Signum  Commented=on
  Terminator1 : Terminator  Commented=on
  Triggered Subsystem1 : Subsystem  Commented=on  TreatAsAtomicUnit=on
  Output : Outport
  wires:
  Clock/1 -> MATLAB Function3/2(t)
  Memory/1 -> MATLAB Function1/2(u1delay)
  Sign/1 -> MATLAB Function1/1(u1), Memory/1
  MATLAB Function1/1(y) -> MATLAB Function3/3(u)
  roadinfo/1 -> MATLAB Function3/1(roadinfo)
  In1/1 -> Sign/1
  param/1 -> MATLAB Function3/4(throshold)
  Relational Operator1/1 -> Logical Operator1/2
  Triggered Subsystem1/2(t3) -> Add1/1
  Enabled Subsystem1/2(t2_laneid) -> Relational Operator1/2
  Compare To Constant2/1 -> Triggered Subsystem1/Trigger
  Add1/1 -> MATLAB Function6/2(t_gap)
  MATLAB Function6/1(y) -> Logical Operator1/1
  MATLAB Function4/1(t1_out) -> Triggered Subsystem1/1(t1_out), Compare To Constant2/1
  Logical Operator1/1 -> ?
  Triggered Subsystem1/3(t1_lanid) -> Relational Operator1/1
  MATLAB Function4/2(l1_out) -> Triggered Subsystem1/3(laneinfo)
  Triggered Subsystem1/1(t1) -> Terminator1/1
  MATLAB Function5/1(y) -> MATLAB Function4/3(u), Compare To Constant3/1
  Memory1/1 -> MATLAB Function5/2(u1delay)
  Clock1/1 -> Enabled Subsystem1/1(t2_out), Triggered Subsystem1/2(t_now), MATLAB Function4/2(t)
  Compare To Constant3/1 -> Enabled Subsystem1/Enable
  Sign1/1 -> MATLAB Function5/1(u1), Memory1/1
  Enabled Subsystem1/1(t2) -> Add1/2
  MATLAB Function3/1(y) -> Output/1

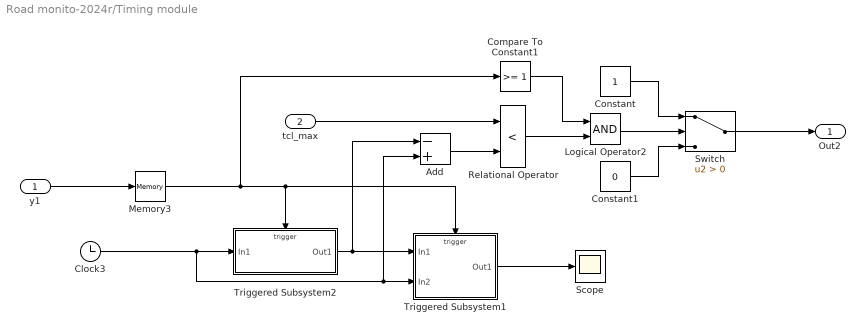
== system Road monito-2024r/Timing module ==
  y1 : Inport
  tcl_max : Inport  Port=2
  Add : Sum  Inputs=-+
  Clock3 : Clock
  Compare To Constant1 : simulink/Logic and Bit Operations/Compare To Constant  relop=>=  const=1  OutDataTypeStr=boolean
  Constant : Constant
  Constant1 : Constant  Value=0
  Logical Operator2 : Logic  AllPortsSameDT=off  OutDataTypeStr=boolean
  Memory3 : Memory
  Relational Operator : RelationalOperator  Operator=<  OutDataTypeStr=boolean  RndMeth=Simplest
  Scope : Scope
  Switch : Switch  Criteria=u2 > Threshold
  Triggered Subsystem1 : Subsystem  TreatAsAtomicUnit=on
  Triggered Subsystem2 : Subsystem  TreatAsAtomicUnit=on
  Out2 : Outport  VectorParamsAs1DForOutWhenUnconnected=off
  wires:
  Relational Operator/1 -> Logical Operator2/2
  Compare To Constant1/1 -> Logical Operator2/1
  Triggered Subsystem1/1(Out1) -> Scope/1
  Logical Operator2/1 -> Switch/2
  y1/1 -> Memory3/1
  Memory3/1 -> Compare To Constant1/1, Triggered Subsystem1/Trigger, Triggered Subsystem2/Trigger
  Add/1 -> Relational Operator/2
  Clock3/1 -> Add/2, Triggered Subsystem1/2(In2), Triggered Subsystem2/1(In1)
  Triggered Subsystem2/1(Out1) -> Add/1, Triggered Subsystem1/1(In1)
  tcl_max/1 -> Relational Operator/1
  Constant/1 -> Switch/1
  Constant1/1 -> Switch/3
  Switch/1 -> Out2/1

== system Road monito-2024r/Triggered Subsystem2 ==
  lane_Ego : Inport
  Trigger : TriggerPort  VariantControl=Variant
  initial : Outport  InitialOutput=0  VectorParamsAs1DForOutWhenUnconnected=off
  wires:
  lane_Ego/1 -> initial/1

== system Road monito-2024r/rule1_1 ==
  Ego : Inport
  Tgtf : Inport  Port=2
  Enable : EnablePort  StatesWhenEnabling=reset
  speed consistent : MATLAB Function  TreatAsAtomicUnit=on
  y : Outport  OutputWhenDisabled=reset  InitialOutput=0
  wires:
  Ego/1 -> speed consistent/1(Ego)
  speed consistent/1(y) -> y/1
  Tgtf/1 -> speed consistent/2(Tgtf)

== system Road monito-2024r/rule1_2_1 ==
  Tgtlf : Inport
  param : Inport  Port=2
  Ego : Inport  Port=3
  Enable : EnablePort  StatesWhenEnabling=reset
  LatDis : MATLAB Function  TreatAsAtomicUnit=on
  y : Outport  OutputWhenDisabled=reset  InitialOutput=0
  wires:
  LatDis/1(y) -> y/1
  Tgtlf/1 -> LatDis/1(Tgtlf)
  Ego/1 -> LatDis/3(Ego)
  param/1 -> LatDis/2(param)

== system Road monito-2024r/rule1_2_2 ==
  Tgtrf : Inport
  param : Inport  Port=2
  Ego : Inport  Port=3
  Enable : EnablePort  StatesWhenEnabling=reset
  LatDis : MATLAB Function  TreatAsAtomicUnit=on
  y : Outport  OutputWhenDisabled=reset  InitialOutput=0
  wires:
  LatDis/1(y) -> y/1
  Tgtrf/1 -> LatDis/1(Tgtrf)
  Ego/1 -> LatDis/3(Ego)
  param/1 -> LatDis/2(param)

== system Road monito-2024r/rule1_2_3 ==
  Tgtlr : Inport
  param : Inport  Port=2
  Ego : Inport  Port=3
  Enable : EnablePort  StatesWhenEnabling=reset
  LatDis : MATLAB Function  TreatAsAtomicUnit=on
  y : Outport  OutputWhenDisabled=reset  InitialOutput=0
  wires:
  LatDis/1(y) -> y/1
  Tgtlr/1 -> LatDis/1(Tgtlr)
  Ego/1 -> LatDis/3(Ego)
  param/1 -> LatDis/2(param)

== system Road monito-2024r/rule1_2_4 ==
  Tgtrr : Inport
  param : Inport  Port=2
  Ego : Inport  Port=3
  Enable : EnablePort  StatesWhenEnabling=reset
  LatDis : MATLAB Function  TreatAsAtomicUnit=on
  y : Outport  OutputWhenDisabled=reset  InitialOutput=0
  wires:
  LatDis/1(y) -> y/1
  Tgtrr/1 -> LatDis/1(Tgtrr)
  Ego/1 -> LatDis/3(Ego)
  param/1 -> LatDis/2(param)

== system Road monito-2024r/rule1_2_5 ==
  Tgtlf : Inport
  param : Inport  Port=2
  Ego : Inport  Port=3
  threshold : Inport  Port=4
  Enable : EnablePort  StatesWhenEnabling=reset
  LatDis : MATLAB Function  TreatAsAtomicUnit=on
  y : Outport  OutputWhenDisabled=reset  InitialOutput=0
  wires:
  LatDis/1(y) -> y/1
  Tgtlf/1 -> LatDis/1(Tgtlf)
  Ego/1 -> LatDis/3(Ego)
  param/1 -> LatDis/2(param)
  threshold/1 -> LatDis/4(threshlod)

== system Road monito-2024r/rule1_2_6 ==
  Tgtrf : Inport
  param : Inport  Port=2
  Ego : Inport  Port=3
  Threshold : Inport  Port=4
  Enable : EnablePort  StatesWhenEnabling=reset
  LatDis : MATLAB Function  TreatAsAtomicUnit=on
  y : Outport  OutputWhenDisabled=reset  InitialOutput=0
  wires:
  LatDis/1(y) -> y/1
  Tgtrf/1 -> LatDis/1(Tgtrf)
  Ego/1 -> LatDis/3(Ego)
  param/1 -> LatDis/2(param)
  Threshold/1 -> LatDis/4(threshlod)

== system Road monito-2024r/rule1_2_7 ==
  Tgtlr : Inport
  param : Inport  Port=2
  Ego : Inport  Port=3
  threshold : Inport  Port=4
  Enable : EnablePort  StatesWhenEnabling=reset
  LatDis : MATLAB Function  TreatAsAtomicUnit=on
  y : Outport  OutputWhenDisabled=reset  InitialOutput=0
  wires:
  LatDis/1(y) -> y/1
  Tgtlr/1 -> LatDis/1(Tgtlr)
  Ego/1 -> LatDis/3(Ego)
  param/1 -> LatDis/2(param)
  threshold/1 -> LatDis/4(threshlod)

== system Road monito-2024r/rule1_2_8 ==
  Tgtrr : Inport
  param : Inport  Port=2
  Ego : Inport  Port=3
  threshold : Inport  Port=4
  Enable : EnablePort  StatesWhenEnabling=reset
  LatDis : MATLAB Function  TreatAsAtomicUnit=on
  y : Outport  OutputWhenDisabled=reset  InitialOutput=0
  wires:
  LatDis/1(y) -> y/1
  Tgtrr/1 -> LatDis/1(Tgtrr)
  Ego/1 -> LatDis/3(Ego)
  param/1 -> LatDis/2(param)
  threshold/1 -> LatDis/4(threshlod)

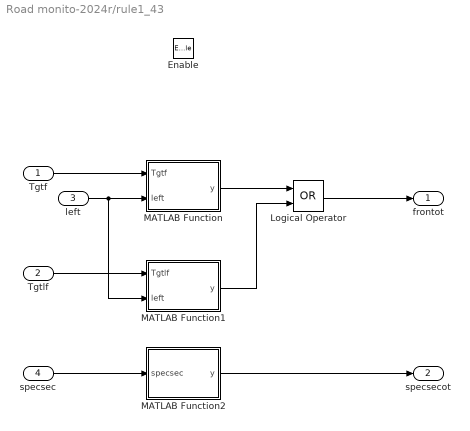
== system Road monito-2024r/rule1_43 ==
  Tgtf : Inport
  Tgtlf : Inport  Port=2
  left : Inport  Port=3
  specsec : Inport  Port=4
  Enable : EnablePort  StatesWhenEnabling=reset
  Logical Operator : Logic  Operator=OR  AllPortsSameDT=off  OutDataTypeStr=boolean
  MATLAB Function : MATLAB Function  TreatAsAtomicUnit=on
  MATLAB Function1 : MATLAB Function  TreatAsAtomicUnit=on
  MATLAB Function2 : MATLAB Function  TreatAsAtomicUnit=on
  frontot : Outport  OutputWhenDisabled=reset  InitialOutput=0
  specsecot : Outport  Port=2  OutputWhenDisabled=reset  InitialOutput=0
  wires:
  Tgtf/1 -> MATLAB Function/1(Tgtf)
  MATLAB Function/1(y) -> Logical Operator/1
  MATLAB Function1/1(y) -> Logical Operator/2
  Logical Operator/1 -> frontot/1
  Tgtlf/1 -> MATLAB Function1/1(Tgtlf)
  left/1 -> MATLAB Function1/2(left), MATLAB Function/2(left)
  specsec/1 -> MATLAB Function2/1(specsec)
  MATLAB Function2/1(y) -> specsecot/1

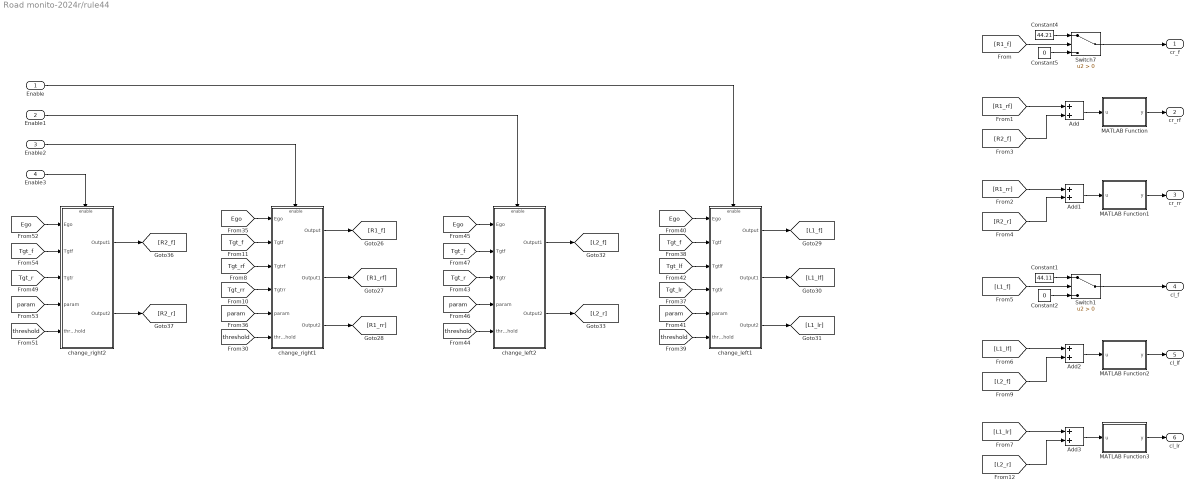
== system Road monito-2024r/rule44 ==
  Enable : Inport
  Enable1 : Inport  Port=2
  Enable2 : Inport  Port=3
  Enable3 : Inport  Port=4
  Add{,1..3} (4 alike) : Sum
  Constant1 : Constant  Value=44.11
  Constant2 : Constant  Value=0
  Constant4 : Constant  Value=44.21
  Constant5 : Constant  Value=0
  MATLAB Function : MATLAB Function  TreatAsAtomicUnit=on
  MATLAB Function1 : MATLAB Function  TreatAsAtomicUnit=on
  MATLAB Function2 : MATLAB Function  TreatAsAtomicUnit=on
  MATLAB Function3 : MATLAB Function  TreatAsAtomicUnit=on
  Switch1 : Switch  Criteria=u2 > Threshold
  Switch7 : Switch  Criteria=u2 > Threshold
  change_left1 : Subsystem  TreatAsAtomicUnit=on
  change_left2 : Subsystem  TreatAsAtomicUnit=on
  change_right1 : Subsystem  TreatAsAtomicUnit=on
  change_right2 : Subsystem  TreatAsAtomicUnit=on
  cr_f : Outport
  cr_rf : Outport  Port=2
  cr_rr : Outport  Port=3
  cl_f : Outport  Port=4
  cl_lf : Outport  Port=5
  cl_lr : Outport  Port=6
  wires:
  [Tgt_f] -> change_right1/2(Tgtf)
  change_right1/2(Output1) -> [R1_rf]
  change_right1/1(Output) -> [R1_f]
  change_left2/2(Output2) -> [L2_r]
  [Tgt_rf] -> change_right1/3(Tgtrf)
  [param] -> change_right1/5(param)
  change_right1/3(Output2) -> [R1_rr]
  [Ego] -> change_right1/1(Ego)
  [Tgt_f] -> change_right2/2(Tgtf)
  [Tgt_rr] -> change_right1/4(Tgtrr)
  change_left1/1(Output) -> [L1_f]
  [Tgt_lf] -> change_left1/3(Tgtlf)
  [param] -> change_left2/4(param)
  Enable/1 -> change_left1/Enable
  change_left1/2(Output1) -> [L1_lf]
  [threshold] -> change_right1/6(threshold)
  [threshold] -> change_left1/6(threshold)
  [param] -> change_right2/4(param)
  change_left2/1(Output1) -> [L2_f]
  change_left1/3(Output2) -> [L1_lr]
  Enable3/1 -> change_right2/Enable
  [Tgt_f] -> change_left1/2(Tgtf)
  Enable1/1 -> change_left2/Enable
  change_right2/1(Output1) -> [R2_f]
  [param] -> change_left1/5(param)
  [Ego] -> change_left1/1(Ego)
  Enable2/1 -> change_right1/Enable
  [threshold] -> change_right2/5(threshold)
  [Tgt_lr] -> change_left1/4(Tgtlr)
  [Tgt_r] -> change_right2/3(Tgtr)
  change_right2/2(Output2) -> [R2_r]
  [Ego] -> change_right2/1(Ego)
  [Ego] -> change_left2/1(Ego)
  [threshold] -> change_left2/5(threshold)
  [Tgt_f] -> change_left2/2(Tgtf)
  [Tgt_r] -> change_left2/3(Tgtr)
  Constant5/1 -> Switch7/3
  Constant4/1 -> Switch7/1
  Switch7/1 -> cr_f/1
  [R1_f] -> Switch7/2
  [R1_rf] -> Add/1
  [R2_f] -> Add/2
  Add/1 -> MATLAB Function/1(u)
  MATLAB Function/1(y) -> cr_rf/1
  MATLAB Function1/1(y) -> cr_rr/1
  Add1/1 -> MATLAB Function1/1(u)
  [R2_r] -> Add1/2
  [R1_rr] -> Add1/1
  MATLAB Function3/1(y) -> cl_lr/1
  Add3/1 -> MATLAB Function3/1(u)
  [L2_f] -> Add2/2
  Add2/1 -> MATLAB Function2/1(u)
  [L1_f] -> Switch1/2
  Constant2/1 -> Switch1/3
  Constant1/1 -> Switch1/1
  MATLAB Function2/1(y) -> cl_lf/1
  [L2_r] -> Add3/2
  [L1_lf] -> Add2/1
  [L1_lr] -> Add3/1
  Switch1/1 -> cl_f/1

== system Road monito-2024r/rule46_1 ==
  Ego : Inport
  Enable : EnablePort  StatesWhenEnabling=reset
  Speedmonitor : MATLAB Function  TreatAsAtomicUnit=on
  y1 : Outport  OutputWhenDisabled=reset  InitialOutput=0
  cs : Outport  Port=2  OutputWhenDisabled=reset  InitialOutput=[0 120]
  wires:
  Speedmonitor/2(cs) -> cs/1
  Ego/1 -> Speedmonitor/1(Ego)
  Speedmonitor/1(y) -> y1/1

== system Road monito-2024r/rule46_2 ==
  Ego : Inport
  Enable : EnablePort  StatesWhenEnabling=reset
  Speedmonitor : MATLAB Function  TreatAsAtomicUnit=on
  y1 : Outport  OutputWhenDisabled=reset  InitialOutput=0
  cs : Outport  Port=2  OutputWhenDisabled=reset  InitialOutput=[0 120]
  wires:
  Speedmonitor/1(y) -> y1/1
  Ego/1 -> Speedmonitor/1(Ego)
  Speedmonitor/2(cs) -> cs/1

== system Road monito-2024r/rule47_1_l ==
  threshold : Inport
  light : Inport  Port=2
  Enable : EnablePort  StatesWhenEnabling=reset
  Speedmonitor : MATLAB Function  TreatAsAtomicUnit=on
  y1 : Outport  OutputWhenDisabled=reset  InitialOutput=0
  wires:
  light/1 -> Speedmonitor/2(light)
  Speedmonitor/1(y) -> y1/1
  threshold/1 -> Speedmonitor/1(threshold)

== system Road monito-2024r/rule47_1_r ==
  threshold : Inport
  light : Inport  Port=2
  Enable : EnablePort  StatesWhenEnabling=reset
  Speedmonitor : MATLAB Function  TreatAsAtomicUnit=on
  y1 : Outport  OutputWhenDisabled=reset  InitialOutput=0
  wires:
  threshold/1 -> Speedmonitor/1(threshold)
  Speedmonitor/1(y) -> y1/1
  light/1 -> Speedmonitor/2(light)

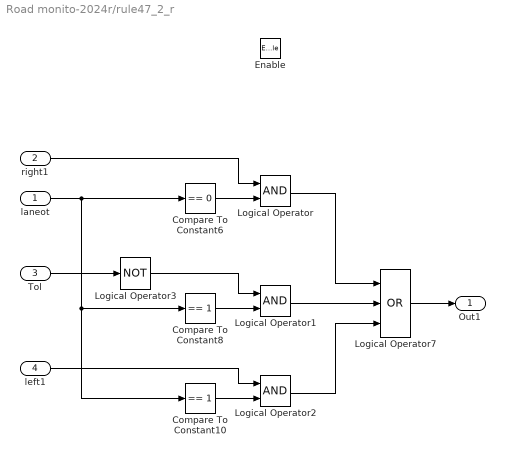
== system Road monito-2024r/rule47_2_r ==
  laneot : Inport
  right1 : Inport  Port=2
  Tol : Inport  Port=3
  left1 : Inport  Port=4
  Enable : EnablePort  StatesWhenEnabling=reset
  Compare To Constant10 : simulink/Logic and Bit Operations/Compare To Constant  relop===  const=1  OutDataTypeStr=boolean
  Compare To Constant6 : simulink/Logic and Bit Operations/Compare To Constant  relop===  const=0  OutDataTypeStr=boolean
  Compare To Constant8 : simulink/Logic and Bit Operations/Compare To Constant  relop===  const=1  OutDataTypeStr=boolean
  Logical Operator : Logic  AllPortsSameDT=off  OutDataTypeStr=boolean
  Logical Operator1 : Logic  AllPortsSameDT=off  OutDataTypeStr=boolean
  Logical Operator2 : Logic  AllPortsSameDT=off  OutDataTypeStr=boolean
  Logical Operator3 : Logic  Operator=NOT  AllPortsSameDT=off  OutDataTypeStr=boolean
  Logical Operator7 : Logic  Operator=OR  Inputs=3  AllPortsSameDT=off  OutDataTypeStr=boolean
  Out1 : Outport  OutputWhenDisabled=reset  InitialOutput=0
  wires:
  Compare To Constant6/1 -> Logical Operator/2
  laneot/1 -> Compare To Constant10/1, Compare To Constant8/1, Compare To Constant6/1
  Compare To Constant8/1 -> Logical Operator1/2
  Compare To Constant10/1 -> Logical Operator2/2
  right1/1 -> Logical Operator/1
  Tol/1 -> Logical Operator3/1
  Logical Operator3/1 -> Logical Operator1/1
  left1/1 -> Logical Operator2/1
  Logical Operator1/1 -> Logical Operator7/2
  Logical Operator/1 -> Logical Operator7/1
  Logical Operator2/1 -> Logical Operator7/3
  Logical Operator7/1 -> Out1/1

== system Road monito-2024r/rule53_1 ==
  In1 : Inport
  Enable : EnablePort  StatesWhenEnabling=reset
  Constant : Constant
  Constant1 : Constant  Value=0
  Switch : Switch  Criteria=u2 > Threshold
  Output : Outport  OutputWhenDisabled=reset  InitialOutput=0
  wires:
  In1/1 -> Switch/2
  Constant/1 -> Switch/1
  Constant1/1 -> Switch/3
  Switch/1 -> Output/1

== system Road monito-2024r/rule58_1 ==
  light : Inport
  Enable : EnablePort  StatesWhenEnabling=reset
  light usage : MATLAB Function  TreatAsAtomicUnit=on
  y : Outport  OutputWhenDisabled=reset  InitialOutput=0
  wires:
  light/1 -> light usage/1(light)
  light usage/1(y) -> y/1

== system Road monito-2024r/rule58_2 ==
  light : Inport
  Enable : EnablePort  StatesWhenEnabling=reset
  light usage : MATLAB Function  TreatAsAtomicUnit=on
  y : Outport  OutputWhenDisabled=reset  InitialOutput=0
  wires:
  light/1 -> light usage/1(light)
  light usage/1(y) -> y/1

== system Road monito-2024r/rule78 ==
  Ego : Inport
  speedsign : Inport  Port=2
  respeedsign : Inport  Port=3
  roadinfo : Inport  Port=4
  Enable : EnablePort  StatesWhenEnabling=reset
  AreaDetermine : Subsystem
  Speedmonitor : MATLAB Function  TreatAsAtomicUnit=on
  Speedsigncalculate : MATLAB Function  TreatAsAtomicUnit=on
  y1 : Outport  OutputWhenDisabled=reset  InitialOutput=0
  y2 : Outport  Port=2  OutputWhenDisabled=reset  InitialOutput=[0 120]
  wires:
  Speedmonitor/1(y) -> y1/1
  Ego/1 -> Speedsigncalculate/1(Ego), Speedmonitor/1(Ego)
  Speedmonitor/3(clear) -> AreaDetermine/2(clear)
  speedsign/1 -> Speedsigncalculate/2(speedsign), Speedmonitor/2(speedsign)
  AreaDetermine/1(spdsign_section) -> Speedmonitor/4(spdsign_section)
  Speedsigncalculate/1(Enter_spdlimit_section) -> AreaDetermine/1(Enter)
  respeedsign/1 -> Speedmonitor/3(respeedsign)
  Speedmonitor/2(cs) -> y2/1
  roadinfo/1 -> Speedmonitor/5(roadinfo)

== system Road monito-2024r/rule79_1 ==
  light : Inport
  Enable : EnablePort  StatesWhenEnabling=reset
  light usage : MATLAB Function  TreatAsAtomicUnit=on
  y : Outport  OutputWhenDisabled=reset  InitialOutput=0
  wires:
  light usage/1(y) -> y/1
  light/1 -> light usage/1(light)

== system Road monito-2024r/rule79_2 ==
  rule44 : Inport
  Enable : EnablePort  StatesWhenEnabling=reset
  Selector : Selector  InputPortWidth=6  IndexOptions=Index vector (dialog)  Indices=[5 6]  OutputSizes=1
  y : Outport  OutputWhenDisabled=reset  InitialOutput=0
  wires:
  Selector/1 -> y/1
  rule44/1 -> Selector/1

== system Road monito-2024r/rule79_3 ==
  light : Inport
  Enable : EnablePort  StatesWhenEnabling=reset
  light usage : MATLAB Function  TreatAsAtomicUnit=on
  y : Outport  OutputWhenDisabled=reset  InitialOutput=0
  wires:
  light/1 -> light usage/1(light)
  light usage/1(y) -> y/1

== system Road monito-2024r/rule79_4 ==
  Ego : Inport
  threshold : Inport  Port=2
  Enable : EnablePort  StatesWhenEnabling=reset
  MATLAB Function : MATLAB Function  TreatAsAtomicUnit=on
  y : Outport  OutputWhenDisabled=reset  InitialOutput=0
  wires:
  MATLAB Function/1(y) -> y/1
  Ego/1 -> MATLAB Function/1(Ego)
  threshold/1 -> MATLAB Function/2(threshold)

== system Road monito-2024r/rule79_5 ==
  Ego : Inport
  threshold : Inport  Port=2
  Enable : EnablePort  StatesWhenEnabling=reset
  MATLAB Function : MATLAB Function  TreatAsAtomicUnit=on
  y : Outport  OutputWhenDisabled=reset  InitialOutput=0
  wires:
  MATLAB Function/1(y) -> y/1
  Ego/1 -> MATLAB Function/1(Ego)
  threshold/1 -> MATLAB Function/2(threshold)

== system Road monito-2024r/rule80 ==
  Ego : Inport
  Enable : EnablePort  StatesWhenEnabling=reset
  FollowingDistance : MATLAB Function  TreatAsAtomicUnit=on
  FollowingDistance1 : MATLAB Function  Commented=on  TreatAsAtomicUnit=on
  CD : Outport  OutputWhenDisabled=reset  InitialOutput=-1
  wires:
  Ego/1 -> FollowingDistance/1(Ego)
  FollowingDistance/1(CD) -> CD/1

== system Road monito-2024r/rule81_1 ==
  light : Inport
  Enable : EnablePort  StatesWhenEnabling=reset
  light usage : MATLAB Function  TreatAsAtomicUnit=on
  y : Outport  OutputWhenDisabled=reset  InitialOutput=0
  wires:
  light/1 -> light usage/1(light)
  light usage/1(y) -> y/1
